simulink model "Concatenate_TestGen11"  (R2017b)
settings: Solver=FixedStepDiscrete  StartTime=0.0  StopTime=10.0  RelTol=1e-3
settings Model: Creator=ktrinh  LastModifiedBy=ktrinh
settings DebuggingCC: ParameterOverflowMsg=none

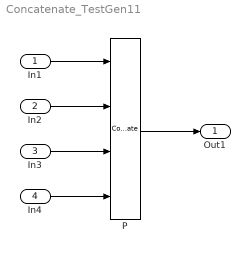
== system Concatenate_TestGen11 ==
  In1 : Inport  OutDataTypeStr=int16  PortDimensions=[3 4 5]
  In2 : Inport  Port=2  OutDataTypeStr=int16  PortDimensions=[3 4 5]
  In3 : Inport  Port=3  OutDataTypeStr=int16  PortDimensions=[3 4 5]
  In4 : Inport  Port=4  OutDataTypeStr=int16  PortDimensions=[3 4 5]
  P : Concatenate  NumInputs=4  Mode=Multidimensional array
  Out1 : Outport
  wires:
  In1/1 -> P/1
  In2/1 -> P/2
  In3/1 -> P/3
  In4/1 -> P/4
  P/1 -> Out1/1
